simulink model "ARDrone2_Comparison"  (R2014b)
settings: Solver=ode45  StartTime=0.0  StopTime=10.0  RelTol=1e-3
settings Model: Creator=m  LastModifiedBy=m

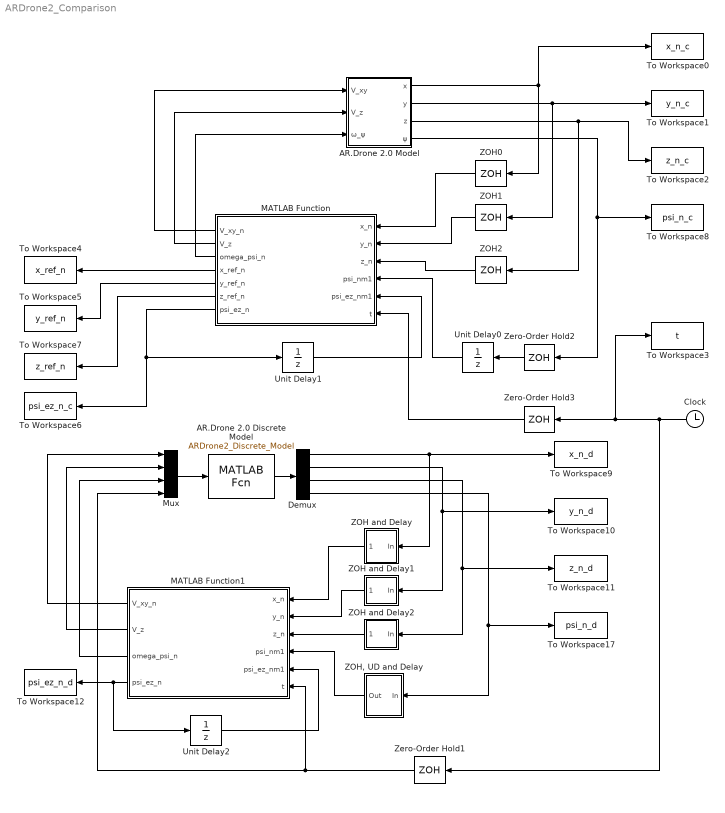
== system ARDrone2_Comparison ==
  AR.Drone 2.0 Discrete Model : MATLABFcn  MATLABFcn=ARDrone2_Discrete_Model  OutputSignalType=real  SampleTime=0.1
  AR.Drone 2.0 Model : Subsystem
  Clock : Clock
  Demux : Demux
  MATLAB Function : MATLAB Function  TreatAsAtomicUnit=on
  MATLAB Function1 : MATLAB Function  TreatAsAtomicUnit=on
  Mux : Mux
  To Workspace0 : ToWorkspace  VariableName=x_n_c  SampleTime=0.1
  To Workspace1 : ToWorkspace  VariableName=y_n_c  SampleTime=0.1
  To Workspace10 : ToWorkspace  VariableName=y_n_d  SampleTime=0.1
  To Workspace11 : ToWorkspace  VariableName=z_n_d  SampleTime=0.1
  To Workspace12 : ToWorkspace  VariableName=psi_ez_n_d  SampleTime=0.1
  To Workspace17 : ToWorkspace  VariableName=psi_n_d  SampleTime=0.1
  To Workspace2 : ToWorkspace  VariableName=z_n_c  SampleTime=0.1
  To Workspace3 : ToWorkspace  VariableName=t  SampleTime=0.1
  To Workspace4 : ToWorkspace  VariableName=x_ref_n  SampleTime=0.1
  To Workspace5 : ToWorkspace  VariableName=y_ref_n  SampleTime=0.1
  To Workspace6 : ToWorkspace  VariableName=psi_ez_n_c  SampleTime=0.1
  To Workspace7 : ToWorkspace  VariableName=z_ref_n  SampleTime=0.1
  To Workspace8 : ToWorkspace  VariableName=psi_n_c  SampleTime=0.1
  To Workspace9 : ToWorkspace  VariableName=x_n_d  SampleTime=0.1
  Unit Delay0 : UnitDelay  SampleTime=-1
  Unit Delay1 : UnitDelay  SampleTime=-1
  Unit Delay2 : UnitDelay  SampleTime=-1
  ZOH and Delay : Subsystem
  ZOH and Delay1 : Subsystem
  ZOH and Delay2 : Subsystem
  "ZOH, UD and Delay" : Subsystem
  ZOH0 : ZeroOrderHold  SampleTime=0.1
  ZOH1 : ZeroOrderHold  SampleTime=0.1
  ZOH2 : ZeroOrderHold  SampleTime=0.1
  Zero-Order Hold1 : ZeroOrderHold  SampleTime=0.1
  Zero-Order Hold2 : ZeroOrderHold  SampleTime=0.1
  Zero-Order Hold3 : ZeroOrderHold  SampleTime=0.1
  wires:
  AR.Drone 2.0 Model/2(y) -> To Workspace1/1, ZOH1/1
  AR.Drone 2.0 Model/4(ψ) -> Zero-Order Hold2/1, To Workspace8/1
  Clock/1 -> Zero-Order Hold1/1, Zero-Order Hold3/1, To Workspace3/1
  AR.Drone 2.0 Model/1(x) -> To Workspace0/1, ZOH0/1
  ZOH0/1 -> MATLAB Function/1(x_n)
  ZOH1/1 -> MATLAB Function/2(y_n)
  Zero-Order Hold2/1 -> Unit Delay0/1
  Unit Delay0/1 -> MATLAB Function/4(psi_nm1)
  Zero-Order Hold3/1 -> MATLAB Function/6(t)
  Unit Delay1/1 -> MATLAB Function/5(psi_ez_nm1)
  MATLAB Function/1(V_xy_n) -> AR.Drone 2.0 Model/1(V_xy)
  MATLAB Function/3(omega_psi_n) -> AR.Drone 2.0 Model/3(ω_ψ)
  MATLAB Function/4(x_ref_n) -> To Workspace4/1
  MATLAB Function/5(y_ref_n) -> To Workspace5/1
  AR.Drone 2.0 Model/3(z) -> ZOH2/1, To Workspace2/1
  ZOH2/1 -> MATLAB Function/3(z_n)
  MATLAB Function/6(z_ref_n) -> To Workspace7/1
  MATLAB Function/7(psi_ez_n) -> Unit Delay1/1, To Workspace6/1
  MATLAB Function/2(V_z) -> AR.Drone 2.0 Model/2(V_z)
  Demux/2 -> ZOH and Delay1/1(In), To Workspace10/1
  Demux/4 -> "ZOH, UD and Delay"/1(In), To Workspace17/1
  Demux/1 -> ZOH and Delay/1(In), To Workspace9/1
  ZOH and Delay1/1(Out) -> MATLAB Function1/2(y_n)
  Zero-Order Hold1/1 -> Mux/4, MATLAB Function1/6(t)
  Unit Delay2/1 -> MATLAB Function1/5(psi_ez_nm1)
  MATLAB Function1/1(V_xy_n) -> Mux/1
  MATLAB Function1/3(omega_psi_n) -> Mux/3
  ZOH and Delay2/1(Out) -> MATLAB Function1/3(z_n)
  MATLAB Function1/4(psi_ez_n) -> To Workspace12/1, Unit Delay2/1
  MATLAB Function1/2(V_z) -> Mux/2
  Mux/1 -> AR.Drone 2.0 Discrete Model/1
  AR.Drone 2.0 Discrete Model/1 -> Demux/1
  Demux/3 -> ZOH and Delay2/1(In), To Workspace11/1
  ZOH and Delay/1(Out) -> MATLAB Function1/1(x_n)
  "ZOH, UD and Delay"/1(Out) -> MATLAB Function1/4(psi_nm1)

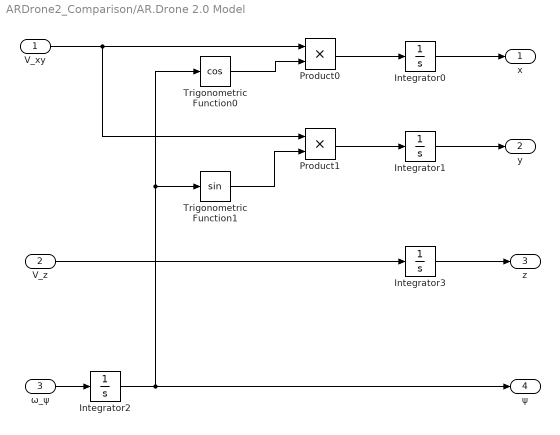
== system ARDrone2_Comparison/AR.Drone 2.0 Model ==
  V_xy : Inport
  V_z : Inport  Port=2
  ω_ψ : Inport  Port=3
  Integrator0 : Integrator
  Integrator1 : Integrator
  Integrator2 : Integrator  InitialCondition=0.01
  Integrator3 : Integrator
  Product0 : Product
  Product1 : Product
  Trigonometric Function0 : Trigonometry  Operator=cos
  Trigonometric Function1 : Trigonometry
  x : Outport
  y : Outport  Port=2
  z : Outport  Port=3
  ψ : Outport  Port=4
  wires:
  Integrator2/1 -> ψ/1, Trigonometric Function0/1, Trigonometric Function1/1
  Product0/1 -> Integrator0/1
  ω_ψ/1 -> Integrator2/1
  V_xy/1 -> Product1/1, Product0/1
  Product1/1 -> Integrator1/1
  Trigonometric Function0/1 -> Product0/2
  Trigonometric Function1/1 -> Product1/2
  Integrator1/1 -> y/1
  Integrator0/1 -> x/1
  Integrator3/1 -> z/1
  V_z/1 -> Integrator3/1

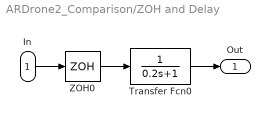
== system ARDrone2_Comparison/ZOH and Delay ==
  In : Inport
  Transfer Fcn0 : TransferFcn  Denominator=[0.2 1]
  ZOH0 : ZeroOrderHold  SampleTime=0.1
  Out : Outport
  wires:
  ZOH0/1 -> Transfer Fcn0/1
  Transfer Fcn0/1 -> Out/1
  In/1 -> ZOH0/1

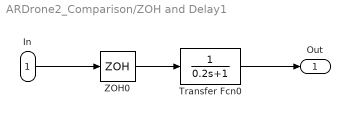
== system ARDrone2_Comparison/ZOH and Delay1 ==
  In : Inport
  Transfer Fcn0 : TransferFcn  Denominator=[0.2 1]
  ZOH0 : ZeroOrderHold  SampleTime=0.1
  Out : Outport
  wires:
  ZOH0/1 -> Transfer Fcn0/1
  Transfer Fcn0/1 -> Out/1
  In/1 -> ZOH0/1

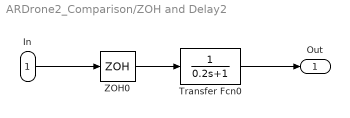
== system ARDrone2_Comparison/ZOH and Delay2 ==
  In : Inport
  Transfer Fcn0 : TransferFcn  Denominator=[0.2 1]
  ZOH0 : ZeroOrderHold  SampleTime=0.1
  Out : Outport
  wires:
  ZOH0/1 -> Transfer Fcn0/1
  Transfer Fcn0/1 -> Out/1
  In/1 -> ZOH0/1

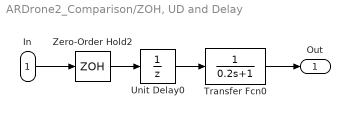
== system ARDrone2_Comparison/ZOH, UD and Delay ==
  In : Inport
  Transfer Fcn0 : TransferFcn  Denominator=[0.2 1]
  Unit Delay0 : UnitDelay  SampleTime=-1
  Zero-Order Hold2 : ZeroOrderHold  SampleTime=0.1
  Out : Outport
  wires:
  Transfer Fcn0/1 -> Out/1
  Unit Delay0/1 -> Transfer Fcn0/1
  In/1 -> Zero-Order Hold2/1
  Zero-Order Hold2/1 -> Unit Delay0/1

== matlab function ARDrone2_Comparison/MATLAB Function1 ==
  data: V_xy_n output; V_z output; omega_psi_n output; x_n input; y_n input; z_n input; psi_nm1 input; psi_ez_nm1 input; t input; psi_ez_n output
%%%%%%%%%%%%%%%%%%%%%%%%%% AR.DRONE 2.0 CONTROLLER %%%%%%%%%%%%%%%%%%%%%%%%
%%%%%%%%%%%%%%%%%%%%%%%%%%%%%%%%%%%%%%%%%%%%%%%%%%%%%%%%%%%%%%%%%%%%%%%%%%%
function [V_xy_n, V_z, omega_psi_n, psi_ez_n]= ...
    controller(x_n, y_n, z_n, psi_nm1, psi_ez_nm1, t)
    
    output = commonController([x_n, y_n, z_n, psi_nm1, psi_ez_nm1, t]);
    V_xy_n = output(1);
    V_z = output(2);
    omega_psi_n = output(3);
    psi_ez_n = output(4);
%%%%%%%%%%%%%%%%%%%%%%%%%%%%%%%%%%%%%%%%%%%%%%%%%%%%%%%%%%%%%%%%%%%%%%%%%%%

== matlab function ARDrone2_Comparison/MATLAB Function ==
  data: V_xy_n output; V_z output; omega_psi_n output; x_ref_n output; y_ref_n output; z_ref_n output; x_n input; y_n input; z_n input; psi_nm1 input; psi_ez_nm1 input; t input; psi_ez_n output
%%%%%%%%%%%%%%%%%%%%%%%%%% AR.DRONE 2.0 CONTROLLER %%%%%%%%%%%%%%%%%%%%%%%%
%%%%%%%%%%%%%%%%%%%%%%%%%%%%%%%%%%%%%%%%%%%%%%%%%%%%%%%%%%%%%%%%%%%%%%%%%%%
function [V_xy_n, V_z, omega_psi_n, x_ref_n, y_ref_n, z_ref_n, psi_ez_n]= ...
    controller(x_n, y_n, z_n, psi_nm1, psi_ez_nm1, t)

    output = commonController([x_n, y_n, z_n, psi_nm1, psi_ez_nm1, t]);
    V_xy_n = output(1);
    V_z = output(2);
    omega_psi_n = output(3);
    psi_ez_n = output(4);
    x_ref_n = output(5);
    y_ref_n = output(6);
    z_ref_n = output(7);
%%%%%%%%%%%%%%%%%%%%%%%%%%%%%%%%%%%%%%%%%%%%%%%%%%%%%%%%%%%%%%%%%%%%%%%%%%%
